simulink model "Merged_model_cost"  (R2022a)
settings: Solver=VariableStepAuto  StartTime=0.0  StopTime=8  RelTol=1e-3
model workspace (MATLAB code in the model file):
  | P1 = [2 0.5 1.6];
  | P2 = [2 -0.5 1.6];
  | P3 = [1.6 0.5 0.9];
  | P4 = [1.6 0 0.9];
  | P5 = [2 0.5 1.6];
  | 
  | t_sim = [0 8];
  | 
  | BlueBase_L = 0.8;
  | BlueBrick_L = 0.3;
  | Red_L = 1.05;
  | Green_L = 0.8;
  | GreenBrick_L = 0.3;
  | White_L = 1.05;
  | LBlue_L = 0.4;
  | Grey_L = 1.175;
  | Black_L = 0.2;
undefined symbols (not defined in the file or in its folder): B, Spline, X, Y, Z
libraries: sm_lib x96, nesl_utility x46, slpidlib x6, robotcorelib x3, simulink_extras x2
(part 1 of 5)
settings Model: Creator=Jakob  LastModifiedBy=Jakob
settings ExplorerConfigSet: InternalSimMechanicsExplorerSettings="<ExplorerConfiguration><canonicalview>default</canonicalview><AnimationSetting><BasePlaybackSpeed>1.0</BasePlaybackSpeed><PlaybackSpeedFactor>1.0</PlaybackSpeedFactor></AnimationSetting><TilePanel><TileInfo><Tiles Columns=\"1\" Count=\"1\" Rows=\"1\"><Column Weight=\"1\"/><Row Weight=\"1\"/><Tile Height=\"1\" Width=\"1\" X=\"0\" Y=\"0\"/></Tiles></TileInfo><SceneInfo><SceneViewer><BGColor><R>0.60000002384185791</R><G>0.60000002384185791</G><B>0.60000002384185791</B></BGColor><Camera><DoPerspective>off</DoPerspective><Position><X>1.65739520996109513</X><Y>-0.87991711964003394</Y><Z>2.2044685892746374</Z></Position><Center><X>0.604268399596188166</X><Y>0.1732096907248728</Y><Z>1.15134177890973088</Z></Center><Up><X>-0.408248290463863073</X><Y>0.408248290463863073</Y><Z>0.816496580927726145</Z></Up><ViewLimDist>1</ViewLimDist><YLim>1.01161623001098633</YLim><XLim>1.3820438478967827</XLim></Camera></SceneViewer></SceneInfo></TilePanel><MechEditorPanel><Cameras/><GfxPanelCameraMap/><VideoCreator><PlaybackSpeedRatio>1.0</PlaybackSpeedRatio><FrameRate>30</FrameRate><VideoFormat>Motion JPEG AVI</VideoFormat><FrameSize>auto</FrameSize></VideoCreator></MechEditorPanel></ExplorerConfiguration>"

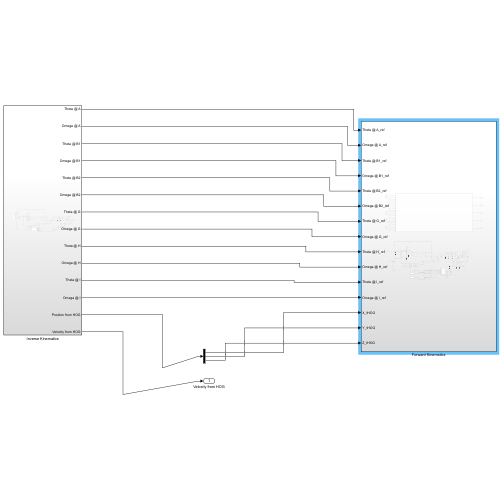
[thumbnail: Simulink's stored preview of the top-level diagram]
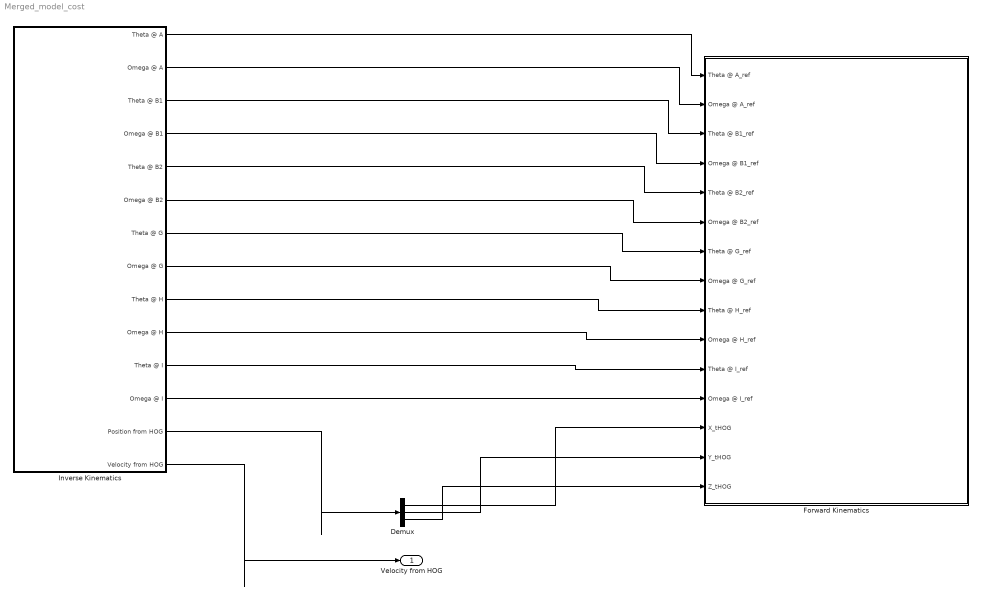
== system Merged_model_cost ==
  Demux : Demux  Outputs=3
  Forward Kinematics : Subsystem
  Inverse Kinematics : Subsystem
  Velocity from HOG : Outport
  wires:
  Inverse Kinematics/1(Theta @ A) -> Forward Kinematics/1(Theta @ A_ref)
  Inverse Kinematics/2(Omega @ A) -> Forward Kinematics/2(Omega @ A_ref)
  Inverse Kinematics/9(Theta @ H) -> Forward Kinematics/9(Theta @ H_ref)
  Inverse Kinematics/10(Omega @ H) -> Forward Kinematics/10(Omega @ H_ref)
  Inverse Kinematics/3(Theta @ B1) -> Forward Kinematics/3(Theta @ B1_ref)
  Inverse Kinematics/4(Omega @ B1) -> Forward Kinematics/4(Omega @ B1_ref)
  Inverse Kinematics/8(Omega @ G) -> Forward Kinematics/8(Omega @ G_ref)
  Inverse Kinematics/7(Theta @ G) -> Forward Kinematics/7(Theta @ G_ref)
  Inverse Kinematics/11(Theta @ I) -> Forward Kinematics/11(Theta @ I_ref)
  Inverse Kinematics/5(Theta @ B2) -> Forward Kinematics/5(Theta @ B2_ref)
  Inverse Kinematics/6(Omega @ B2) -> Forward Kinematics/6(Omega @ B2_ref)
  Inverse Kinematics/13(Position from HOG) -> Demux/1
  Inverse Kinematics/12(Omega @ I) -> Forward Kinematics/12(Omega @ I_ref)
  Inverse Kinematics/14(Velocity from HOG) -> Velocity from HOG/1
  Demux/1 -> Forward Kinematics/13(X_tHOG)
  Demux/2 -> Forward Kinematics/14(Y_tHOG)
  Demux/3 -> Forward Kinematics/15(Z_tHOG)
